simulink model "untitled"  (R2017a)
settings: Solver=FixedStepDiscrete  StartTime=0.0  StopTime=inf  RelTol=1e-3
undefined symbols (not defined in the file): N, serial
libraries: simulink x4, instrumentlib x3
settings Model: Creator=VarvaR  LastModifiedBy=VarvaR

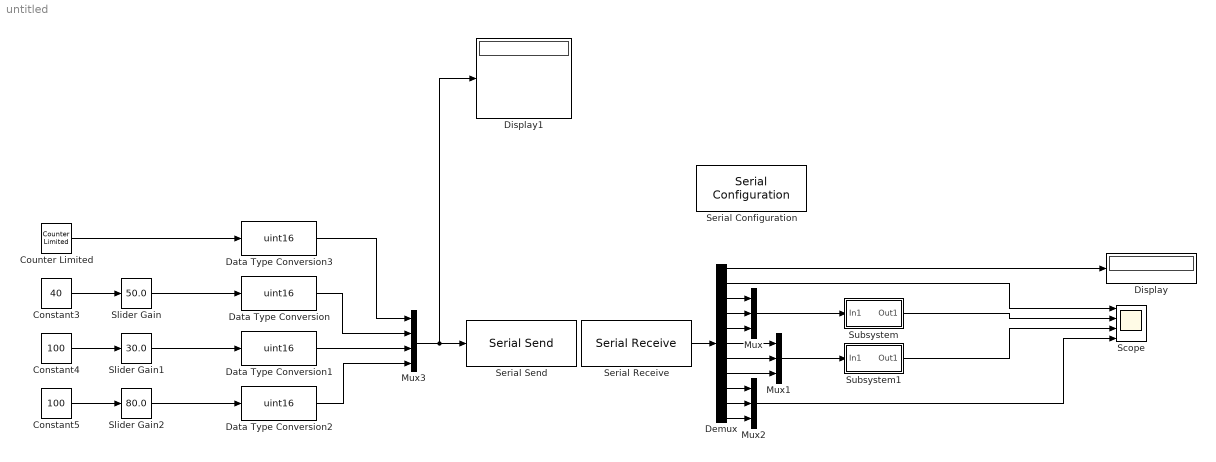
== system untitled ==
  Constant3 : Constant  Value=40  SampleTime=0.1
  Constant4 : Constant  Value=100  SampleTime=0.1
  Constant5 : Constant  Value=100  SampleTime=0.1
  Counter Limited : simulink/Sources/Counter Limited  uplimit=10  tsamp=0.1
  Data Type Conversion{,1..3} (4 alike) : DataTypeConversion  OutDataTypeStr=uint16
  Demux : Demux  Outputs=11
  Display : Display
      settings: Format=hex (Stored Integer)
  Display1 : Display
      settings: Format=hex (Stored Integer)
  Mux : Mux  Inputs=3
  Mux1 : Mux  Inputs=3
  Mux2 : Mux  Inputs=3
  Mux3 : Mux
  Scope : Scope  NumInputPorts=4
  Serial Configuration : instrumentlib/Serial Configuration  Priority=-200000  ComPortMenu=COM8  ComPort=COM8  ObjConstructor=serial('COM8');  BaudRate=10000000  DataBits=8  Parity=none  StopBits=1  FlowControl=none  Timeout=10  ByteOrder=LittleEndian
  Serial Receive : instrumentlib/Serial Receive  ComPortMenu=COM8  ComPort=COM8  ObjConstructor=serial('COM8');  Terminator=<none>  DataSize="[1  11]"  DataType=uint16  EnableBlockingMode=on  ActionDataUnavailable=Output last received value  CustomValue=0  SampleTime=0.01
  Serial Send : instrumentlib/Serial Send  ComPortMenu=COM8  ComPort=COM8  ObjConstructor=serial('COM8');  Header=7F7A  Terminator=<none>  EnableBlockingMode=on
  Slider Gain : simulink/Math Operations/Slider Gain  gain=50.0  low=0  high=100
  Slider Gain1 : simulink/Math Operations/Slider Gain  gain=30.0  low=0  high=100
  Slider Gain2 : simulink/Math Operations/Slider Gain  gain=80.0  low=0  high=100
  Subsystem : Subsystem
  Subsystem1 : Subsystem
  wires:
  Serial Receive/1 -> Demux/1
  Mux/1 -> Subsystem/1(In1)
  Subsystem/1(Out1) -> Scope/2
  Demux/2 -> Scope/1
  Demux/3 -> Mux/1
  Demux/4 -> Mux/2
  Demux/5 -> Mux/3
  Demux/8 -> Mux1/3
  Demux/7 -> Mux1/2
  Demux/6 -> Mux1/1
  Demux/10 -> Mux2/2
  Demux/11 -> Mux2/3
  Demux/9 -> Mux2/1
  Mux1/1 -> Subsystem1/1(In1)
  Subsystem1/1(Out1) -> Scope/3
  Mux2/1 -> Scope/4
  Demux/1 -> Display/1
  Constant5/1 -> Slider Gain2/1
  Slider Gain/1 -> Data Type Conversion/1
  Data Type Conversion3/1 -> Mux3/1
  Data Type Conversion2/1 -> Mux3/4
  Slider Gain1/1 -> Data Type Conversion1/1
  Data Type Conversion/1 -> Mux3/2
  Constant4/1 -> Slider Gain1/1
  Slider Gain2/1 -> Data Type Conversion2/1
  Constant3/1 -> Slider Gain/1
  Counter Limited/1 -> Data Type Conversion3/1
  Data Type Conversion1/1 -> Mux3/3
  Mux3/1 -> Display1/1, Serial Send/1

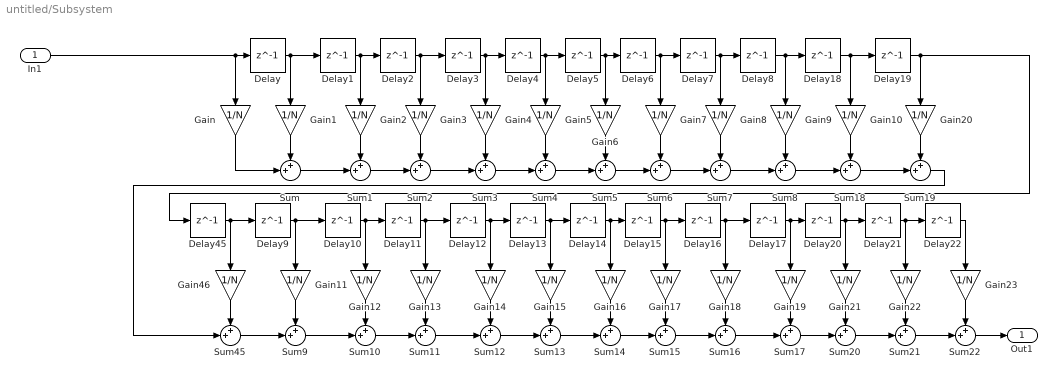
== system untitled/Subsystem ==
  In1 : Inport
  Delay{,1..22,45} (24 alike) : Delay  DelayLength=1
  Gain{,1..23,46} (25 alike) : Gain  Gain=1/N
  Sum{,1..22,45} (24 alike) : Sum  Inputs=++|
  Out1 : Outport
  wires:
  Delay/1 -> Delay1/1, Gain1/1
  Gain1/1 -> Sum/1
  Gain/1 -> Sum/2
  In1/1 -> Delay/1, Gain/1
  Gain2/1 -> Sum1/1
  Delay1/1 -> Delay2/1, Gain2/1
  Gain3/1 -> Sum2/1
  Delay2/1 -> Delay3/1, Gain3/1
  Gain4/1 -> Sum3/1
  Delay3/1 -> Delay4/1, Gain4/1
  Gain5/1 -> Sum4/1
  Delay4/1 -> Delay5/1, Gain5/1
  Gain6/1 -> Sum5/1
  Delay5/1 -> Delay6/1, Gain6/1
  Gain7/1 -> Sum6/1
  Delay6/1 -> Delay7/1, Gain7/1
  Gain8/1 -> Sum7/1
  Delay7/1 -> Delay8/1, Gain8/1
  Gain9/1 -> Sum8/1
  Sum7/1 -> Sum8/2
  Sum6/1 -> Sum7/2
  Sum5/1 -> Sum6/2
  Sum4/1 -> Sum5/2
  Sum3/1 -> Sum4/2
  Sum2/1 -> Sum3/2
  Sum1/1 -> Sum2/2
  Sum/1 -> Sum1/2
  Gain12/1 -> Sum10/1
  Delay15/1 -> Delay16/1, Gain17/1
  Gain17/1 -> Sum15/1
  Delay12/1 -> Delay13/1, Gain14/1
  Sum10/1 -> Sum11/2
  Gain15/1 -> Sum13/1
  Sum11/1 -> Sum12/2
  Gain14/1 -> Sum12/1
  Delay16/1 -> Delay17/1, Gain18/1
  Gain18/1 -> Sum16/1
  Delay13/1 -> Delay14/1, Gain15/1
  Sum13/1 -> Sum14/2
  Gain11/1 -> Sum9/1
  Sum9/1 -> Sum10/2
  Sum14/1 -> Sum15/2
  Gain13/1 -> Sum11/1
  Sum12/1 -> Sum13/2
  Delay10/1 -> Delay11/1, Gain12/1
  Sum15/1 -> Sum16/2
  Delay14/1 -> Delay15/1, Gain16/1
  Gain16/1 -> Sum14/1
  Gain19/1 -> Sum17/1
  Sum16/1 -> Sum17/2
  Delay11/1 -> Delay12/1, Gain13/1
  Delay9/1 -> Delay10/1, Gain11/1
  Delay8/1 -> Gain9/1, Delay18/1
  Sum19/1 -> Sum45/2
  Delay17/1 -> Delay20/1, Gain19/1
  Gain46/1 -> Sum45/1
  Sum45/1 -> Sum9/2
  Delay45/1 -> Gain46/1, Delay9/1
  Delay18/1 -> Delay19/1, Gain10/1
  Gain10/1 -> Sum18/1
  Sum8/1 -> Sum18/2
  Delay19/1 -> Delay45/1, Gain20/1
  Gain20/1 -> Sum19/1
  Sum18/1 -> Sum19/2
  Gain21/1 -> Sum20/1
  Sum17/1 -> Sum20/2
  Delay20/1 -> Delay21/1, Gain21/1
  Gain22/1 -> Sum21/1
  Sum20/1 -> Sum21/2
  Delay21/1 -> Delay22/1, Gain22/1
  Gain23/1 -> Sum22/1
  Sum21/1 -> Sum22/2
  Delay22/1 -> Gain23/1
  Sum22/1 -> Out1/1

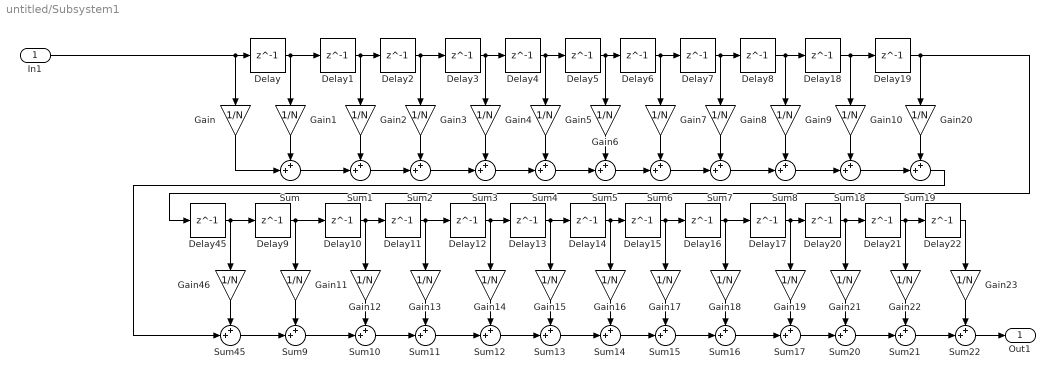
== system untitled/Subsystem1 ==
  In1 : Inport
  Delay{,1..22,45} (24 alike) : Delay  DelayLength=1
  Gain{,1..23,46} (25 alike) : Gain  Gain=1/N
  Sum{,1..22,45} (24 alike) : Sum  Inputs=++|
  Out1 : Outport
  wires:
  Delay/1 -> Delay1/1, Gain1/1
  Gain1/1 -> Sum/1
  Gain/1 -> Sum/2
  In1/1 -> Delay/1, Gain/1
  Gain2/1 -> Sum1/1
  Delay1/1 -> Delay2/1, Gain2/1
  Gain3/1 -> Sum2/1
  Delay2/1 -> Delay3/1, Gain3/1
  Gain4/1 -> Sum3/1
  Delay3/1 -> Delay4/1, Gain4/1
  Gain5/1 -> Sum4/1
  Delay4/1 -> Delay5/1, Gain5/1
  Gain6/1 -> Sum5/1
  Delay5/1 -> Delay6/1, Gain6/1
  Gain7/1 -> Sum6/1
  Delay6/1 -> Delay7/1, Gain7/1
  Gain8/1 -> Sum7/1
  Delay7/1 -> Delay8/1, Gain8/1
  Gain9/1 -> Sum8/1
  Sum7/1 -> Sum8/2
  Sum6/1 -> Sum7/2
  Sum5/1 -> Sum6/2
  Sum4/1 -> Sum5/2
  Sum3/1 -> Sum4/2
  Sum2/1 -> Sum3/2
  Sum1/1 -> Sum2/2
  Sum/1 -> Sum1/2
  Gain12/1 -> Sum10/1
  Delay15/1 -> Delay16/1, Gain17/1
  Gain17/1 -> Sum15/1
  Delay12/1 -> Delay13/1, Gain14/1
  Sum10/1 -> Sum11/2
  Gain15/1 -> Sum13/1
  Sum11/1 -> Sum12/2
  Gain14/1 -> Sum12/1
  Delay16/1 -> Delay17/1, Gain18/1
  Gain18/1 -> Sum16/1
  Delay13/1 -> Delay14/1, Gain15/1
  Sum13/1 -> Sum14/2
  Gain11/1 -> Sum9/1
  Sum9/1 -> Sum10/2
  Sum14/1 -> Sum15/2
  Gain13/1 -> Sum11/1
  Sum12/1 -> Sum13/2
  Delay10/1 -> Delay11/1, Gain12/1
  Sum15/1 -> Sum16/2
  Delay14/1 -> Delay15/1, Gain16/1
  Gain16/1 -> Sum14/1
  Gain19/1 -> Sum17/1
  Sum16/1 -> Sum17/2
  Delay11/1 -> Delay12/1, Gain13/1
  Delay9/1 -> Delay10/1, Gain11/1
  Delay8/1 -> Gain9/1, Delay18/1
  Sum19/1 -> Sum45/2
  Delay17/1 -> Delay20/1, Gain19/1
  Gain46/1 -> Sum45/1
  Sum45/1 -> Sum9/2
  Delay45/1 -> Gain46/1, Delay9/1
  Delay18/1 -> Delay19/1, Gain10/1
  Gain10/1 -> Sum18/1
  Sum8/1 -> Sum18/2
  Delay19/1 -> Delay45/1, Gain20/1
  Gain20/1 -> Sum19/1
  Sum18/1 -> Sum19/2
  Gain21/1 -> Sum20/1
  Sum17/1 -> Sum20/2
  Delay20/1 -> Delay21/1, Gain21/1
  Gain22/1 -> Sum21/1
  Sum20/1 -> Sum21/2
  Delay21/1 -> Delay22/1, Gain22/1
  Gain23/1 -> Sum22/1
  Sum21/1 -> Sum22/2
  Delay22/1 -> Gain23/1
  Sum22/1 -> Out1/1
